simulink model "q_servo_pos_cntrl2"  (R2019a)
settings: Solver=ode4  StartTime=0.0  StopTime=inf  FixedStep=0.002  RelTol=1e-3
values from neighbouring files (symbols this model uses):
  kd = 0    [setup_servo_pos_cntrl2.m]
  ki = 0    [setup_servo_pos_cntrl2.m]
  kp = 0    [setup_servo_pos_cntrl2.m]
undefined symbols (not defined in the file or in its folder): HIL, K_ENC, qc_get_step_size, VMAX_DAC
libraries: quarc_library x4
settings Model: ExtModeTrigDuration=10000  Creator=MLevis  LastModifiedBy=pmartin
settings DataIOCC: ReturnWorkspaceOutputs=off
settings DebuggingCC: UnderspecifiedInitializationDetection=Classic  MergeDetectMultiDrivingBlocksExec=none
settings ModelReferenceCC: PropagateSignalLabelsOutOfModel=off

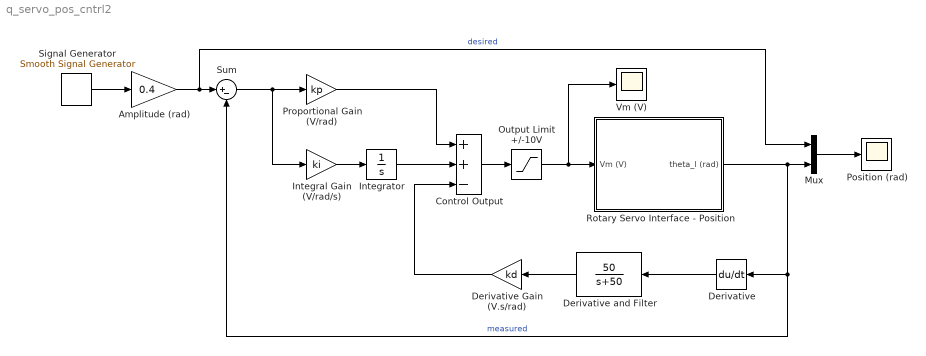
== system q_servo_pos_cntrl2 ==
  Amplitude (rad) : Gain  Gain=0.4  SaturateOnIntegerOverflow=on  OutDataTypeStr=Inherit: Same as input  ParamDataTypeStr=Inherit: Same as input
  Control Output : Sum  Inputs=++-
  Derivative : Derivative
  Derivative Gain (V.s/rad) : Gain  Gain=kd
  Derivative and Filter : TransferFcn  Numerator=[50]  Denominator=[1 50]
  Integral Gain (V/rad/s) : Gain  Gain=ki
  Integrator : Integrator  UpperSaturationLimit=VMAX_DAC  LowerSaturationLimit=-VMAX_DAC
  Mux : Mux  Inputs=2
  Output Limit +/-10V : Saturate  UpperLimit=10  LowerLimit=-10
  Position (rad) : Scope
  Proportional Gain (V/rad) : Gain  Gain=kp
  Rotary Servo Interface - Position : Subsystem
  Signal Generator : quarc_library/Sources/Signals/Smooth Signal Generator  signal_type=Square  source=Internal (dialog parameters)  amplitude=1  frequency=0.4  initial_phase=0  sample_time=qc_get_step_size  output_cos=off
      settings: SourceProductName=QUARC Targets
  Sum : Sum  Inputs=|+-
  Vm (V) : Scope
  wires:
  Signal Generator/1 -> Amplitude (rad)/1
  Rotary Servo Interface - Position/1(theta_l (rad)) -> Derivative/1, Sum/2, Mux/2  "measured"
  Integrator/1 -> Control Output/2
  Mux/1 -> Position (rad)/1
  Derivative Gain (V.s/rad)/1 -> Control Output/3
  Sum/1 -> Integral Gain (V/rad/s)/1, Proportional Gain (V/rad)/1
  Control Output/1 -> Output Limit +/-10V/1
  Integral Gain (V/rad/s)/1 -> Integrator/1
  Proportional Gain (V/rad)/1 -> Control Output/1
  Output Limit +/-10V/1 -> Vm (V)/1, Rotary Servo Interface - Position/1(Vm (V))
  Amplitude (rad)/1 -> Mux/1, Sum/1  "desired"
  Derivative and Filter/1 -> Derivative Gain (V.s/rad)/1
  Derivative/1 -> Derivative and Filter/1

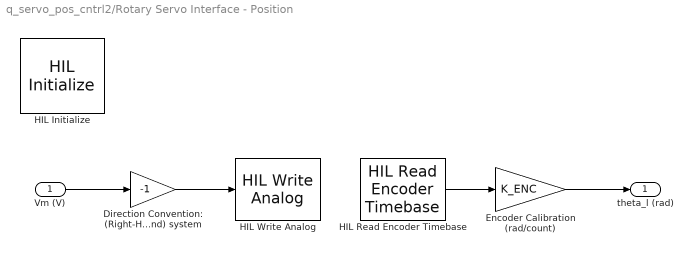
== system q_servo_pos_cntrl2/Rotary Servo Interface - Position ==
  Vm (V) : Inport
  Direction Convention: (Right-Hand) system : Gain  Gain=-1  SaturateOnIntegerOverflow=on  OutDataTypeStr=Inherit: Same as input  ParamDataTypeStr=Inherit: Same as input
  Encoder Calibration (rad/count) : Gain  Gain=K_ENC  SaturateOnIntegerOverflow=on  OutDataTypeStr=Inherit: Same as input  ParamDataTypeStr=Inherit: Same as input
  HIL Initialize : quarc_library/Data Acquisition/Generic/Configuration/HIL Initialize  object_name=HIL-1  board_type=q8_usb  board_number=0@tcpip://localhost:18940  board_options=update_rate=normal;decimation=1  exclusive=off  active=on  hardware_clocks=[0:2]  clock_modes=[]  initial_clock_frequencies=[]  set_clock_params_at_start=off  set_clock_params_at_switch_in=off  set_clock_frequencies_at_start=off  set_clock_frequencies_at_switch_in=off  analog_input_channels=[0:7]  analog_input_configurations=[]  analog_input_maximums=10  analog_input_minimums=-10  set_analog_input_params_at_start=on  set_analog_input_params_at_switch_in=off  analog_output_channels=[0:7]  analog_output_maximums=10  analog_output_minimums=-10  initial_analog_outputs=[0]  final_analog_outputs=[0]  watchdog_analog_outputs=0  set_analog_output_params_at_start=on  set_analog_output_params_at_switch_in=off  set_analog_outputs_at_start=on  set_analog_outputs_at_switch_in=off  set_analog_outputs_at_terminate=on  set_analog_outputs_at_switch_out=off  set_analog_outputs_on_watchdog=off  digital_input_channels=[]  digital_output_channels=[]  digital_output_configuration=[]  initial_digital_outputs=[1]  final_digital_outputs=[1]  watchdog_digital_outputs=[1]  set_digital_output_params_at_start=off  set_digital_output_params_at_switch_in=off  set_digital_outputs_at_start=on  set_digital_outputs_at_switch_in=off  set_digital_outputs_at_terminate=on  set_digital_outputs_at_switch_out=off  set_digital_outputs_on_watchdog=off  encoder_channels=[0:7]  quadrature=[4]  encoder_filter_frequency=[]  initial_encoder_counts=[0]  set_encoder_params_at_start=on  set_encoder_params_at_switch_in=off  set_encoder_counts_at_start=on  set_encoder_counts_at_switch_in=off  pwm_channels=[0:7]  pwm_modes=0  pwm_frequency=99.532799999999995e6/4095  pwm_configuration=[0]  pwm_alignment=[0]  pwm_polarity=[1]  pwm_leading_deadband=[0]  pwm_trailing_deadband=[0]  initial_pwm_outputs=[0]  final_pwm_outputs=[0]  watchdog_pwm_outputs=[0]  set_pwm_params_at_start=on  set_pwm_params_at_switch_in=off  set_pwm_outputs_at_start=on  set_pwm_outputs_at_switch_in=off  set_pwm_outputs_at_terminate=on  set_pwm_outputs_at_switch_out=off  set_pwm_outputs_on_watchdog=off  other_output_channels=[]  initial_other_outputs=[]  final_other_outputs=[]  watchdog_other_outputs=[]  set_other_outputs_at_start=off  set_other_outputs_at_switch_in=off  set_other_outputs_at_terminate=off  set_other_outputs_at_switch_out=off  set_other_outputs_on_watchdog=off
  HIL Read Encoder Timebase : quarc_library/Data Acquisition/Generic/Timebases/HIL Read Encoder Timebase  object_name=HIL-1  clock=0  channels=0  active=on  vector_output=off  data_type_mode=Inherit via back propagation  data_type=double  overflow_mode=Synchronize (for simulated cards only)  samples_in_buffer=1 + 0 * max(ceil(1/qc_get_step_size), 1)
  HIL Write Analog : quarc_library/Data Acquisition/Generic/Immediate I//O/HIL Write Analog  Tag=unassigned  object_name=HIL-1  channels=0  sample_time=-1  active=on  vector_input=off
  theta_l (rad) : Outport
  wires:
  Vm (V)/1 -> Direction Convention: (Right-Hand) system/1
  Direction Convention: (Right-Hand) system/1 -> HIL Write Analog/1
  Encoder Calibration (rad/count)/1 -> theta_l (rad)/1
  HIL Read Encoder Timebase/1 -> Encoder Calibration (rad/count)/1
